simulink model "ROSCO_v1"  (R2023a)
settings: Solver=ode4  StartTime=0.0  StopTime=TMax  FixedStep=simu.dt  RelTol=1e-3  EnableMultiTasking=on
undefined symbols (not defined in the file): Azimuth_list, DiscIntNeverNeededParam, F, n_FixFrameInputs, n_FixFrameOutputs, n_RotTripletInputs, n_RotTripletOutputs, new_seq_inp, new_seq_out, OutList, Parameter, R, rpm2radps, simu, StateSpace, strmatch
libraries: simulink x10
(part 1 of 3)
settings Model: Creator=nabbas  LastModifiedBy=16708
settings SolverCC: AlgebraicLoopSolver=TrustRegion
settings DataIOCC: SaveTime=off  ReturnWorkspaceOutputs=off  SignalLoggingName=sigsOut
settings DebuggingCC: UnconnectedInputMsg=warning  UnconnectedOutputMsg=warning  UnconnectedLineMsg=warning  ArithmeticOperatorsInVariantConditions=warning
settings ModelReferenceCC: EnableRefExpFcnMdlSchedulingChecks=on
settings SFSimCC: SimUseLocalCustomCode=off  CustomCodeUndefinedFunction=UseInterfaceOnly
settings RTWCC: RTWUseLocalCustomCode=off
settings CodeAppCC: StateflowObjectComments=on

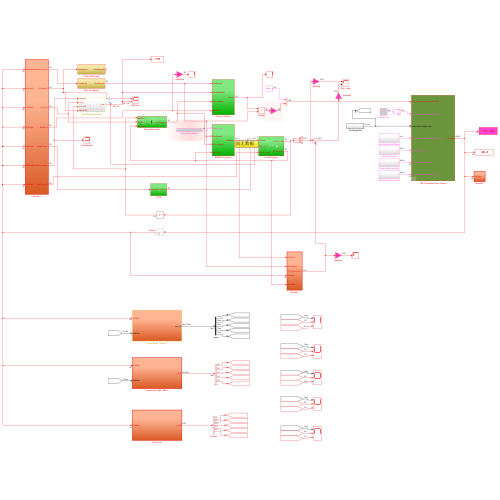
[thumbnail: Simulink's stored preview of the top-level diagram]
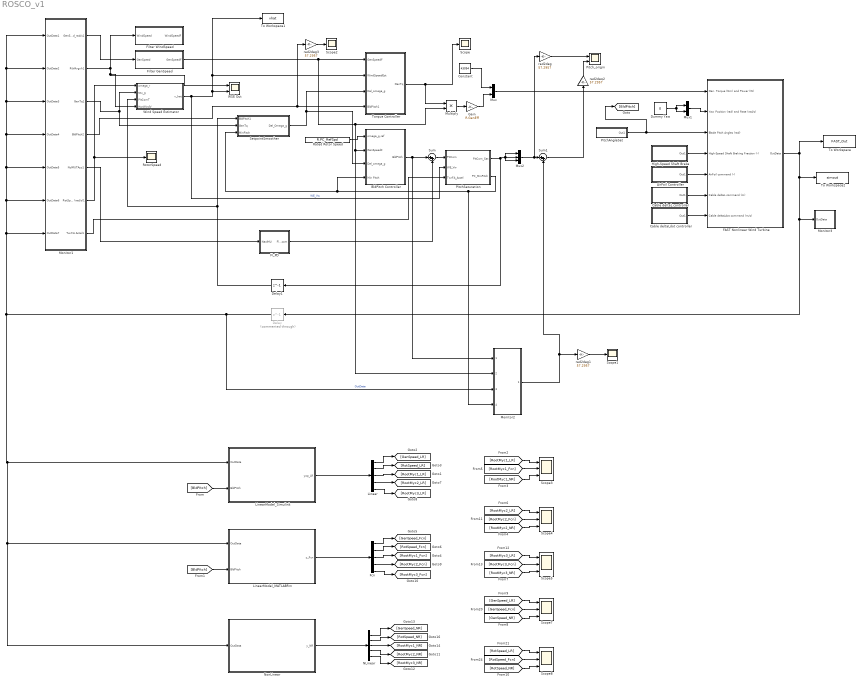
== system ROSCO_v1 ==
  AirFoil Controller : Subsystem
  BldPitch Controller : Subsystem
  Cable deltaL controller : Subsystem
  Cable deltaLdot controller : Subsystem
  Constant : Constant  Value=43094
  Delay : Delay  Commented=through  DelayLength=1
  Delay1 : Delay  DelayLength=1
  Dummy Yaw : Constant  Value=0
  FAST Nonlinear Wind Turbine : Subsystem  mask(FAST Nonlinear Wind Turbine){}
      mask help: This block contains the FAST S-Function.
      mask init:
      | clear FAST_SFunc
  Fcn : Demux  Outputs=5
  Filter GenSpeed : Subsystem
  Filter WindSpeed : Subsystem
  Fl_PD : Subsystem
  Gain : Gain  Gain=R.GenEff
  High-Speed Shaft Brake : Subsystem
  Linear : Demux  Outputs=5
  LinearModel_MATLABFcn : Subsystem  TreatAsAtomicUnit=on
  LinearModel_Simulink : Subsystem  TreatAsAtomicUnit=on
  Monitor1 : Subsystem  TreatAsAtomicUnit=on
  Monitor2 : Subsystem  TreatAsAtomicUnit=on
  Monitor3 : Subsystem  TreatAsAtomicUnit=on
  Multiply : Product
  Mux : Mux  Inputs=2
  Mux1 : Mux  Inputs=2
  Mux2 : Mux  Inputs=3
  NLinear : Demux  Outputs=5
  NonLinear : Subsystem  TreatAsAtomicUnit=on
  PitchAngleSet : Subsystem
  PitchSaturation : Subsystem
  Pitch_origin : Scope  NumInputPorts=2
  Rated Rotor Speed : Constant  Value=R.PC_RefSpd
  RotorSpeed : Scope
  Scope : Scope
  Scope1 : Scope
  Scope2 : Scope
  Scope{3..5,7..8} (5 alike) : Scope  NumInputPorts=3
  SetpointSmoother : Subsystem
  Sum : Sum  Inputs=|++
  Sum1 : Sum  Inputs=|++
  To Workspace : ToWorkspace  VariableName=FAST_Out  SaveFormat=Timeseries  SampleTime=-1
  To Workspace1 : ToWorkspace  VariableName=vhat  SaveFormat=Timeseries  SampleTime=-1
  To Workspace2 : ToWorkspace  VariableName=simout  SaveFormat=Timeseries  SampleTime=-1
  Torque Controller : Subsystem
  WSE Out : Scope  NumInputPorts=2
  Wind Speed Estimator : Subsystem
  rad2deg{,1..3} (4 alike) : Gain  Gain=57.2957
  wires:
  FAST Nonlinear Wind Turbine/1(OutData) -> To Workspace/1, To Workspace2/1, Monitor3/1(OutData), Delay/1
  Dummy Yaw/1 -> Mux1/2, Mux1/1
  Mux1/1 -> FAST Nonlinear Wind Turbine/2(Yaw Position (rad) and Rate (rad/s))
  Multiply/1 -> Gain/1
  Monitor1/1(GenSpeed_rad/s1) -> Filter GenSpeed/1(GenSpeed)
  Torque Controller/1(GenTq) -> Scope/1, Multiply/1
  Monitor1/3(GenTq1) -> Wind Speed Estimator/2(tau_g), SetpointSmoother/2(GenTq)
  SetpointSmoother/1(Del_Omega_g) -> BldPitch Controller/3(Del_omega_g), Torque Controller/3(Del_omega_g)
  Rated Rotor Speed/1 -> BldPitch Controller/1(omega_g,ref)
  Gain/1 -> Mux/2
  Monitor1/2(RtVAvgxh1) -> Filter WindSpeed/1(WindSpeed), Wind Speed Estimator/4(HorWindV), WSE Out/1
  Wind Speed Estimator/1(v_hat) -> PitchSaturation/2(WE_Vw), WSE Out/2, Torque Controller/2(WindSpeedEst), To Workspace1/1  "WE_Vw"
  Delay/1 -> Monitor2/3(OutData), NonLinear/1(OutData), LinearModel_MATLABFcn/1(OutData), LinearModel_Simulink/1(OutData), Monitor1/7(OutData7), Monitor1/6(OutData6), Monitor1/5(OutData5), Monitor1/4(OutData4), Monitor1/3(OutData3), Monitor1/1(OutData1), Monitor1/2(OutData2)  "OutData"
  Monitor1/5(NcIMUTAys1) -> Fl_PD/1(NacIMU)
  Fl_PD/1(Fl_Pitcom) -> Sum/2
  Monitor1/4(BldPitch2) -> rad2deg3/1, Torque Controller/4(BldPitch1)
  Sum/1 -> PitchSaturation/1(PitCom)
  PitchSaturation/1(PitCom_Sat) -> Delay1/1, Mux2/3, Mux2/1, Mux2/2
  PitchSaturation/2(PC_MinPitch) -> Monitor2/4(Min Pitch), BldPitch Controller/4(Min Pitch), SetpointSmoother/3(MinPitch)
  BldPitch Controller/1(BldPitch) -> Monitor2/1(Coll.Pitch), Sum/1
  Monitor1/6(RotSpeed (rad/s)1) -> RotorSpeed/1, Wind Speed Estimator/1(omega_r)
  Delay1/1 -> SetpointSmoother/1(BldPitch1), Wind Speed Estimator/3(PitComT)
  Monitor1/7(TwrFA Accel1) -> PitchSaturation/3(TwrFA_Accel)
  Mux/1 -> FAST Nonlinear Wind Turbine/1(Gen. Torque (Nm) and Power (W))
  Filter GenSpeed/1(GenSpeedF) -> Torque Controller/1(GenSpeedF), Multiply/2, Monitor2/2(Gen Speed), BldPitch Controller/2(GenSpeedF)
  Mux2/1 -> rad2deg/1, Sum1/1
  Sum1/1 -> rad2deg2/1
  High-Speed Shaft Brake/1(Out1) -> FAST Nonlinear Wind Turbine/4(High-Speed Shaft Braking Fraction (-))
  AirFoil Controller/1(Out1) -> FAST Nonlinear Wind Turbine/5(AirFoil command (-))
  Cable deltaL controller/1(Out1) -> FAST Nonlinear Wind Turbine/6(Cable deltaL command (m))
  Cable deltaLdot controller/1(Out1) -> FAST Nonlinear Wind Turbine/7(Cable deltaLdot command (m/s))
  rad2deg/1 -> Pitch_origin/1
  Monitor2/1(IPC Cmd (rad,3)) -> rad2deg1/1, Sum1/2
  rad2deg1/1 -> Scope1/1
  rad2deg2/1 -> Pitch_origin/2
  Constant/1 -> Mux/1
  rad2deg3/1 -> Scope2/1
  [BldPitch] -> LinearModel_Simulink/2(BldPitch)
  [BldPitch] -> LinearModel_MATLABFcn/2(BldPitch)
  LinearModel_Simulink/1(yop_LR) -> Linear/1
  Linear/5 -> [RootMyc3_LR]
  Linear/3 -> [RootMyc1_LR]
  Linear/2 -> [RotSpeed_LR]
  Linear/4 -> [RootMyc2_LR]
  Linear/1 -> [GenSpeed_LR]
  Fcn/4 -> [RootMyc2_Fcn]
  Fcn/1 -> [GenSpeed_Fcn]
  Fcn/3 -> [RootMyc1_Fcn]
  LinearModel_MATLABFcn/1(y_Fcn) -> Fcn/1
  Fcn/5 -> [RootMyc3_Fcn]
  Fcn/2 -> [RotSpeed_Fcn]
  [RootMyc2_LR] -> Scope4/1
  [RootMyc3_Fcn] -> Scope5/2
  [RotSpeed_LR] -> Scope8/1
  [GenSpeed_LR] -> Scope7/1
  [RootMyc2_Fcn] -> Scope4/2
  [GenSpeed_Fcn] -> Scope7/2
  [RootMyc1_Fcn] -> Scope3/2
  [RootMyc3_LR] -> Scope5/1
  [RotSpeed_Fcn] -> Scope8/2
  [RootMyc1_LR] -> Scope3/1
  NLinear/3 -> [RootMyc1_NR]
  NonLinear/1(y_NR) -> NLinear/1
  NLinear/5 -> [RootMyc3_NR]
  NLinear/2 -> [RotSpeed_NR]
  NLinear/4 -> [RootMyc2_NR]
  NLinear/1 -> [GenSpeed_NR]
  [RootMyc1_NR] -> Scope3/3
  [RootMyc2_NR] -> Scope4/3
  [RootMyc3_NR] -> Scope5/3
  [GenSpeed_NR] -> Scope7/3
  [RotSpeed_NR] -> Scope8/3
  PitchAngleSet/1(Out1) -> [BldPitch], FAST Nonlinear Wind Turbine/3(Blade Pitch Angles (rad))

== system ROSCO_v1/AirFoil Controller ==
  Airfoil command : Constant  Value=zeros(1,3)'
  Out1 : Outport
  wires:
  Airfoil command/1 -> Out1/1

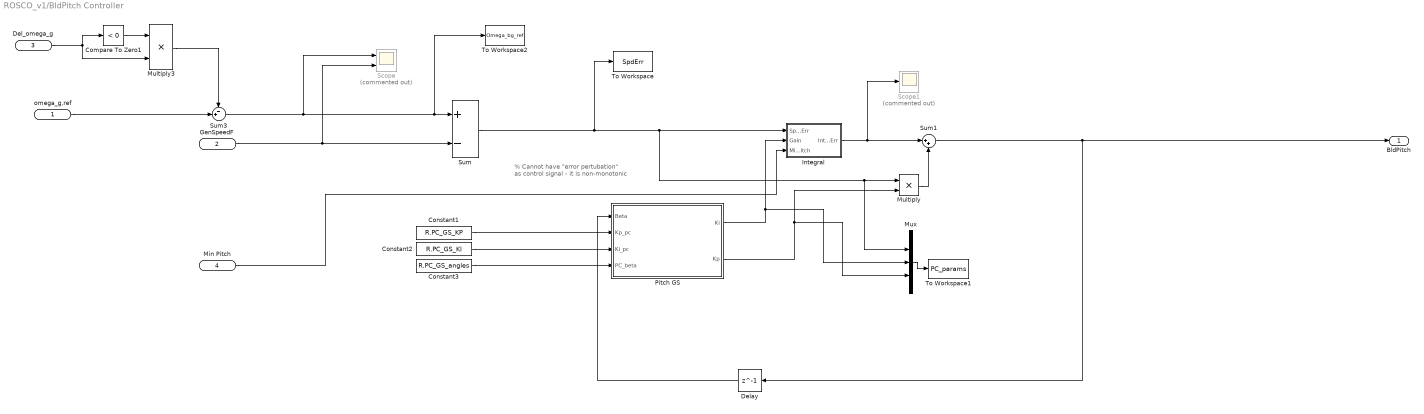
== system ROSCO_v1/BldPitch Controller ==
  note: % Cannot have "error pertubation" as control signal
      | - it is non-monotonic
  omega_g,ref : Inport
  GenSpeedF : Inport  Port=2
  Del_omega_g : Inport  Port=3
  Min Pitch : Inport  Port=4
  Compare To Zero1 : simulink/Logic and Bit Operations/Compare To Zero  relop=<  OutDataTypeStr=boolean
  Constant1 : Constant  Value=R.PC_GS_KP
  Constant2 : Constant  Value=R.PC_GS_KI
  Constant3 : Constant  Value=R.PC_GS_angles
  Delay : Delay  DelayLength=1
  Integral : Subsystem
  Multiply : Product
  Multiply3 : Product
  Mux : Mux  Inputs=5
  Pitch GS : MATLAB Function  TreatAsAtomicUnit=on
  Scope : Scope  Commented=on  NumInputPorts=2
  Scope1 : Scope  Commented=on
  Sum : Sum  Inputs=+-
  Sum1 : Sum  Inputs=|++
  Sum3 : Sum  Inputs=-+|
  To Workspace : ToWorkspace  VariableName=SpdErr  SaveFormat=Timeseries  SampleTime=-1
  To Workspace1 : ToWorkspace  VariableName=PC_params  SaveFormat=Structure  SampleTime=-1
  To Workspace2 : ToWorkspace  VariableName=Omega_bg_ref  SaveFormat=Timeseries  SampleTime=-1
  BldPitch : Outport  VectorParamsAs1DForOutWhenUnconnected=off
  wires:
  Multiply/1 -> Sum1/2
  Integral/1(IntSpdErr) -> Scope1/1, Sum1/1
  Pitch GS/1(Ki) -> Mux/3, Integral/2(Gain)
  Pitch GS/2(Kp) -> Mux/4, Multiply/2
  Mux/1 -> To Workspace1/1
  Sum1/1 -> Delay/1, BldPitch/1
  Sum3/1 -> Scope/1, To Workspace2/1, Sum/1
  GenSpeedF/1 -> Scope/2, Sum/2
  Compare To Zero1/1 -> Multiply3/1
  Del_omega_g/1 -> Compare To Zero1/1, Multiply3/2
  Multiply3/1 -> Sum3/1
  omega_g,ref/1 -> Sum3/2
  Constant1/1 -> Pitch GS/2(Kp_pc)
  Constant2/1 -> Pitch GS/3(Ki_pc)
  Constant3/1 -> Pitch GS/4(PC_beta)
  Delay/1 -> Pitch GS/1(Beta)
  Min Pitch/1 -> Integral/3(Min Pitch)
  Sum/1 -> To Workspace/1, Mux/2, Multiply/1, Integral/1(SpeedErr)

== system ROSCO_v1/Cable deltaL controller ==
  Cable deltaL command : Constant  Value=zeros(1,20)'
  Out1 : Outport
  wires:
  Cable deltaL command/1 -> Out1/1

== system ROSCO_v1/Cable deltaLdot controller ==
  Cable deltaLdot command : Constant  Value=zeros(1,20)'
  Out1 : Outport
  wires:
  Cable deltaLdot command/1 -> Out1/1

== system ROSCO_v1/FAST Nonlinear Wind Turbine ==
  Gen. Torque (Nm) and Power (W) : Inport
  Yaw Position (rad) and Rate (rad/s) : Inport  Port=2
  Blade Pitch Angles (rad) : Inport  Port=3
  High-Speed Shaft Braking Fraction (-) : Inport  Port=4
  AirFoil command (-) : Inport  Port=5
  Cable deltaL command (m) : Inport  Port=6
  Cable deltaLdot command (m/s) : Inport  Port=7
  Mux1 : Mux  Inputs=7
  S-Function : S-Function  FunctionName=FAST_SFunc  Parameters=FAST_InputFileName, TMax, 0  SFunctionDeploymentMode=off  EnableBusSupport=off
  Signal Specification1 : SignalSpecification  OutDataTypeStr=double  Dimensions=2
  Signal Specification2 : SignalSpecification  OutDataTypeStr=double  Dimensions=2
  OutData : Outport
  wires:
  Gen. Torque (Nm) and Power (W)/1 -> Signal Specification1/1
  S-Function/1 -> OutData/1
  Mux1/1 -> S-Function/1
  Blade Pitch Angles (rad)/1 -> Mux1/3
  Yaw Position (rad) and Rate (rad/s)/1 -> Signal Specification2/1
  Signal Specification1/1 -> Mux1/1
  Signal Specification2/1 -> Mux1/2
  High-Speed Shaft Braking Fraction (-)/1 -> Mux1/4
  AirFoil command (-)/1 -> Mux1/5
  Cable deltaL command (m)/1 -> Mux1/6
  Cable deltaLdot command (m/s)/1 -> Mux1/7

== system ROSCO_v1/Filter GenSpeed ==
  GenSpeed : Inport
  Discrete Filter : DiscreteFilter  Numerator=F.HSS.b  Denominator=F.HSS.a  InitialStates=R.VS_RefSpd/(sum(F.HSS.a(2:end))+1)
  Scope : Scope  NumInputPorts=2
  To Workspace2 : ToWorkspace  VariableName=Om_f  SaveFormat=Timeseries  SampleTime=-1
  GenSpeedF : Outport  VectorParamsAs1DForOutWhenUnconnected=off
  wires:
  Discrete Filter/1 -> Scope/2, To Workspace2/1, GenSpeedF/1
  GenSpeed/1 -> Scope/1, Discrete Filter/1

== system ROSCO_v1/Filter WindSpeed ==
  WindSpeed : Inport
  Discrete Filter : DiscreteFilter  Numerator=F.Wind.b  Denominator=F.Wind.a  InitialStates=10
  To Workspace2 : ToWorkspace  VariableName=WindSpeedF  SaveFormat=Timeseries  SampleTime=-1
  WindSpeedF : Outport  VectorParamsAs1DForOutWhenUnconnected=off
  wires:
  Discrete Filter/1 -> WindSpeedF/1, To Workspace2/1
  WindSpeed/1 -> Discrete Filter/1

== system ROSCO_v1/Fl_PD ==
  NacIMU : Inport
  Constant : Constant
  Enable : Gain  Gain=R.Fl_Mode
  Fl_HPF : DiscreteFilter  Numerator=F.F_Fl_HPF.b  Denominator=F.F_Fl_HPF.b
  Fl_LPF : DiscreteFilter  Numerator=F.F_Fl.b  Denominator=F.F_Fl.a
  Gain1 : Gain  Gain=-R.Fl_Kp
  Integral : Subsystem
  Scope : Scope
  Fl_Pitcom : Outport
  wires:
  Constant/1 -> Integral/2(Gain)
  NacIMU/1 -> Fl_LPF/1  "FA_AccR"
  Integral/1(Int x) -> Gain1/1
  Fl_HPF/1 -> Integral/1(x)  "FA_AccF"
  Gain1/1 -> Enable/1  "Fl_Pitcom"
  Enable/1 -> Scope/1, Fl_Pitcom/1  "Fl_Pitcom"
  Fl_LPF/1 -> Fl_HPF/1  "FA_AccF"

== system ROSCO_v1/High-Speed Shaft Brake ==
  High-Speed Shaft Braking Fraction : Constant  Value=0
  Out1 : Outport
  wires:
  High-Speed Shaft Braking Fraction/1 -> Out1/1

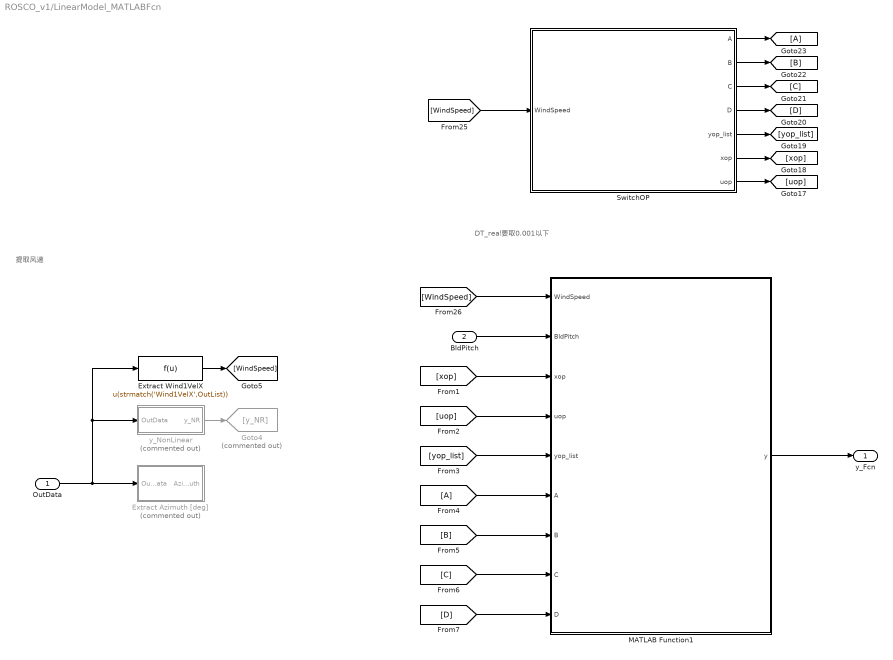
== system ROSCO_v1/LinearModel_MATLABFcn ==
  note: DT_real要取0.001以下
  note: 提取风速
  OutData : Inport
  BldPitch : Inport  Port=2
  Extract Azimuth [deg] : Subsystem  Commented=on
  Extract Wind1VelX : Fcn  Expr=u(strmatch('Wind1VelX',OutList))
  From4 : From
  Goto23 : Goto
  Goto4 : Goto  Commented=on  GotoTag=y_NR
  MATLAB Function1 : MATLAB Function  TreatAsAtomicUnit=on
  SwitchOP : Subsystem
  y_NonLinear : Subsystem  Commented=on
  y_Fcn : Outport
  wires:
  Extract Wind1VelX/1 -> [WindSpeed]
  y_NonLinear/1(y_NR) -> Goto4/1
  OutData/1 -> Extract Azimuth [deg]/1(OutData), y_NonLinear/1(OutData), Extract Wind1VelX/1
  BldPitch/1 -> MATLAB Function1/2(BldPitch)
  [WindSpeed] -> MATLAB Function1/1(WindSpeed)
  [xop] -> MATLAB Function1/3(xop)
  [uop] -> MATLAB Function1/4(uop)
  [yop_list] -> MATLAB Function1/5(yop_list)
  From4/1 -> MATLAB Function1/6(A)
  [B] -> MATLAB Function1/7(B)
  [C] -> MATLAB Function1/8(C)
  [D] -> MATLAB Function1/9(D)
  MATLAB Function1/1(y) -> y_Fcn/1
  SwitchOP/2(B) -> [B]
  SwitchOP/3(C) -> [C]
  SwitchOP/5(yop_list) -> [yop_list]
  SwitchOP/4(D) -> [D]
  SwitchOP/7(uop) -> [uop]
  SwitchOP/1(A) -> Goto23/1
  SwitchOP/6(xop) -> [xop]
  [WindSpeed] -> SwitchOP/1(WindSpeed)

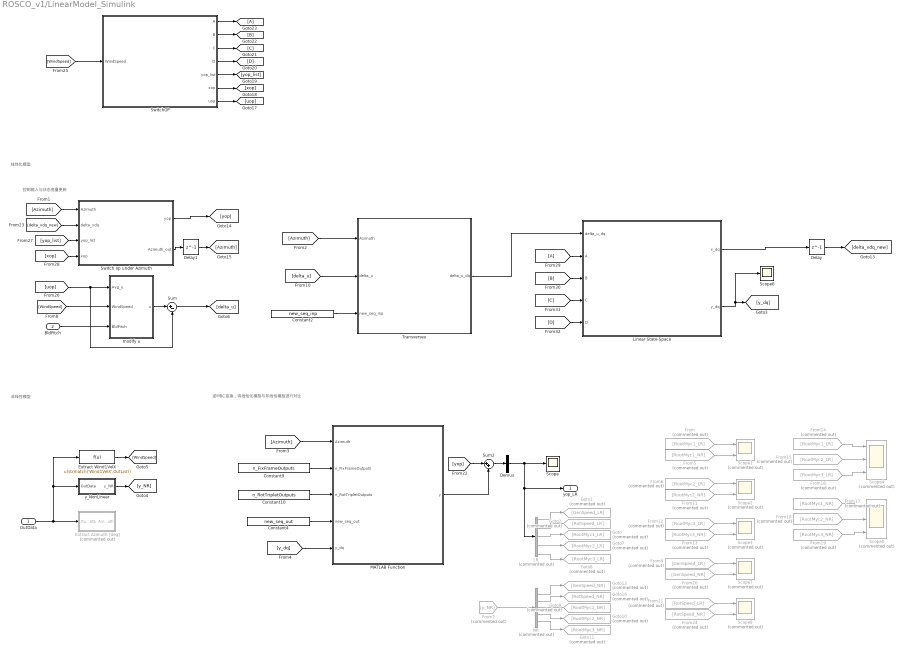
== system ROSCO_v1/LinearModel_Simulink ==
  note: 逆MBC变换，将线性化模型与非线性模型进行对比
  note: 控制输入与状态变量更新
  note: 线性化模型
  note: 非线性模型
  OutData : Inport
  BldPitch : Inport  Port=2
  Constant10 : Constant  Value=n_RotTripletOutputs
  Constant2 : Constant  Value=new_seq_inp
  Constant4 : Constant  Value=new_seq_out
  Constant9 : Constant  Value=n_FixFrameOutputs
  Delay : Delay  DelayLength=1  InitialCondition=0
  Delay1 : Delay  DelayLength=1  InitialCondition=0
  Demux : Demux  Outputs=1
  Extract Azimuth [deg] : Subsystem  Commented=on
  Extract Wind1VelX : Fcn  Expr=u(strmatch('Wind1VelX',OutList))
  From : From  Commented=on  GotoTag=RootMyc1_LR
  From11 : From  Commented=on  GotoTag=RootMyc2_NR
  From12 : From  Commented=on  GotoTag=RootMyc3_LR
  From13 : From  Commented=on  GotoTag=RootMyc3_NR
  From14 : From  Commented=on  GotoTag=RootMyc1_LR
  From15 : From  Commented=on  GotoTag=RootMyc2_LR
  From16 : From  Commented=on  GotoTag=RootMyc3_LR
  From17 : From  Commented=on  GotoTag=RootMyc1_NR
  From18 : From  Commented=on  GotoTag=RootMyc2_NR
  From19 : From  Commented=on  GotoTag=RootMyc3_NR
  From20 : From  Commented=on  GotoTag=GenSpeed_NR
  From21 : From  Commented=on  GotoTag=RotSpeed_LR
  From24 : From  Commented=on  GotoTag=RotSpeed_NR
  From29 : From
  From5 : From  Commented=on  GotoTag=RootMyc1_NR
  From6 : From  Commented=on  GotoTag=RootMyc2_LR
  From7 : From  Commented=on  GotoTag=y_NR
  From9 : From  Commented=on  GotoTag=GenSpeed_LR
  Goto : Goto  Commented=on  GotoTag=RootMyc1_LR
  Goto1 : Goto  Commented=on  GotoTag=GenSpeed_LR
  Goto10 : Goto  Commented=on  GotoTag=RootMyc2_NR
  Goto11 : Goto  Commented=on  GotoTag=RootMyc3_NR
  Goto12 : Goto  Commented=on  GotoTag=GenSpeed_NR
  Goto16 : Goto  Commented=on  GotoTag=RotSpeed_NR
  Goto2 : Goto  Commented=on  GotoTag=RotSpeed_LR
  Goto23 : Goto
  Goto7 : Goto  Commented=on  GotoTag=RootMyc2_LR
  Goto8 : Goto  Commented=on  GotoTag=RootMyc3_LR
  Goto9 : Goto  Commented=on  GotoTag=RootMyc1_NR
  LR : Demux  Commented=on  Outputs=5
  Linear State-Space : Subsystem
  MATLAB Function : MATLAB Function  TreatAsAtomicUnit=on
  NR : Demux  Commented=on  Outputs=5
  Scope : Scope
  Scope{1..3,7..8} (5 alike) : Scope  Commented=on  NumInputPorts=2
  Scope4 : Scope  Commented=on  NumInputPorts=3
  Scope5 : Scope  Commented=on  NumInputPorts=3
  Scope6 : Scope
  Sum : Sum  Inputs=|+-
  Sum2 : Sum  Inputs=|++
  Switch op under Azimuth : Subsystem
  SwitchOP : Subsystem
  Transverseu : Subsystem
  modify u : MATLAB Function  TreatAsAtomicUnit=on
  y_NonLinear : Subsystem
  yop_LR : Outport
  wires:
  OutData/1 -> Extract Wind1VelX/1, y_NonLinear/1(OutData), Extract Azimuth [deg]/1(OutData)
  Transverseu/1(delta_u_dq) -> Linear State-Space/1(delta_u_dq)
  Demux/1 -> Scope/1, yop_LR/1, LR/1
  y_NonLinear/1(y_NR) -> [y_NR]
  From7/1 -> NR/1
  Extract Wind1VelX/1 -> [WindSpeed]
  [Azimuth] -> Transverseu/1(Azimuth)
  Sum/1 -> [delta_u]
  [WindSpeed] -> modify u/2(WindSpeed)
  [uop] -> Sum/2, modify u/1(Avg_u)
  modify u/1(u) -> Sum/1
  [delta_u] -> Transverseu/2(delta_u)
  Constant2/1 -> Transverseu/3(new_seq_inp)
  Constant9/1 -> MATLAB Function/2(n_FixFrameOutputs)
  Constant10/1 -> MATLAB Function/3(n_RotTripletOutputs)
  [Azimuth] -> MATLAB Function/1(Azimuth)
  Constant4/1 -> MATLAB Function/4(new_seq_out)
  [y_dq] -> MATLAB Function/5(y_dq)
  LR/3 -> Goto/1
  LR/4 -> Goto7/1
  LR/5 -> Goto8/1
  NR/3 -> Goto9/1
  NR/4 -> Goto10/1
  NR/5 -> Goto11/1
  From/1 -> Scope1/1
  From5/1 -> Scope1/2
  From6/1 -> Scope2/1
  From11/1 -> Scope2/2
  From12/1 -> Scope3/1
  From13/1 -> Scope3/2
  From14/1 -> Scope4/1
  From15/1 -> Scope4/2
  From16/1 -> Scope4/3
  From17/1 -> Scope5/1
  From18/1 -> Scope5/2
  From19/1 -> Scope5/3
  Linear State-Space/1(x_dq) -> Delay/1
  Switch op under Azimuth/1(yop) -> [yop]
  [Azimuth] -> Switch op under Azimuth/1(Azimuth)
  [yop] -> Sum2/1
  Sum2/1 -> Demux/1
  Linear State-Space/2(y_dq) -> Scope6/1, [y_dq]
  MATLAB Function/1(y) -> Sum2/2
  Delay/1 -> [delta_xdq_new]
  Switch op under Azimuth/2(Azimuth_out) -> Delay1/1
  Delay1/1 -> [Azimuth]
  [delta_xdq_new] -> Switch op under Azimuth/2(delta_xdq)
  LR/1 -> Goto1/1
  LR/2 -> Goto2/1
  NR/1 -> Goto12/1
  NR/2 -> Goto16/1
  From9/1 -> Scope7/1
  From20/1 -> Scope7/2
  From21/1 -> Scope8/1
  From24/1 -> Scope8/2
  BldPitch/1 -> modify u/3(BldPitch)
  [WindSpeed] -> SwitchOP/1(WindSpeed)
  SwitchOP/7(uop) -> [uop]
  SwitchOP/6(xop) -> [xop]
  SwitchOP/5(yop_list) -> [yop_list]
  SwitchOP/4(D) -> [D]
  SwitchOP/3(C) -> [C]
  SwitchOP/2(B) -> [B]
  SwitchOP/1(A) -> Goto23/1
  [yop_list] -> Switch op under Azimuth/3(yop_list)
  [xop] -> Switch op under Azimuth/4(xop)
  From29/1 -> Linear State-Space/2(A)
  [B] -> Linear State-Space/3(B)
  [C] -> Linear State-Space/4(C)
  [D] -> Linear State-Space/5(D)

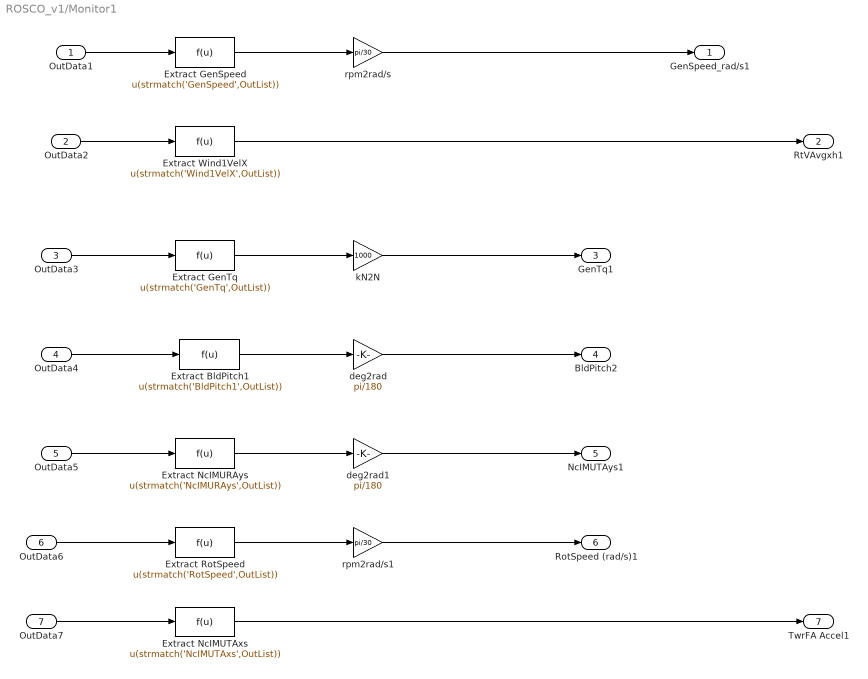
== system ROSCO_v1/Monitor1 ==
  OutData1 : Inport
  OutData2 : Inport  Port=2
  OutData3 : Inport  Port=3
  OutData4 : Inport  Port=4
  OutData5 : Inport  Port=5
  OutData6 : Inport  Port=6
  OutData7 : Inport  Port=7
  Extract BldPitch1 : Fcn  Expr=u(strmatch('BldPitch1',OutList))
  Extract GenSpeed : Fcn  Expr=u(strmatch('GenSpeed',OutList))
  Extract GenTq : Fcn  Expr=u(strmatch('GenTq',OutList))
  Extract NcIMURAys : Fcn  Expr=u(strmatch('NcIMURAys',OutList))
  Extract NcIMUTAxs : Fcn  Expr=u(strmatch('NcIMUTAxs',OutList))
  Extract RotSpeed : Fcn  Expr=u(strmatch('RotSpeed',OutList))
  Extract Wind1VelX : Fcn  Expr=u(strmatch('Wind1VelX',OutList))
  deg2rad : Gain  Gain=pi/180
  deg2rad1 : Gain  Gain=pi/180
  kN2N : Gain  Gain=1000
  rpm2rad/s : Gain  Gain=pi/30
  rpm2rad/s1 : Gain  Gain=pi/30
  GenSpeed_rad/s1 : Outport  VectorParamsAs1DForOutWhenUnconnected=off
  RtVAvgxh1 : Outport  Port=2  VectorParamsAs1DForOutWhenUnconnected=off
  GenTq1 : Outport  Port=3  VectorParamsAs1DForOutWhenUnconnected=off
  BldPitch2 : Outport  Port=4  VectorParamsAs1DForOutWhenUnconnected=off
  NcIMUTAys1 : Outport  Port=5  VectorParamsAs1DForOutWhenUnconnected=off
  RotSpeed (rad/s)1 : Outport  Port=6  VectorParamsAs1DForOutWhenUnconnected=off
  TwrFA Accel1 : Outport  Port=7  VectorParamsAs1DForOutWhenUnconnected=off
  wires:
  Extract NcIMURAys/1 -> deg2rad1/1
  Extract GenSpeed/1 -> rpm2rad/s/1
  OutData5/1 -> Extract NcIMURAys/1
  Extract NcIMUTAxs/1 -> TwrFA Accel1/1
  rpm2rad/s1/1 -> RotSpeed (rad/s)1/1
  Extract RotSpeed/1 -> rpm2rad/s1/1
  Extract BldPitch1/1 -> deg2rad/1
  OutData4/1 -> Extract BldPitch1/1
  rpm2rad/s/1 -> GenSpeed_rad/s1/1
  OutData3/1 -> Extract GenTq/1
  deg2rad1/1 -> NcIMUTAys1/1
  kN2N/1 -> GenTq1/1
  OutData7/1 -> Extract NcIMUTAxs/1
  deg2rad/1 -> BldPitch2/1
  OutData2/1 -> Extract Wind1VelX/1
  Extract GenTq/1 -> kN2N/1
  Extract Wind1VelX/1 -> RtVAvgxh1/1
  OutData1/1 -> Extract GenSpeed/1
  OutData6/1 -> Extract RotSpeed/1

== system ROSCO_v1/Monitor2 ==
  Coll.Pitch : Inport
  Gen Speed : Inport  Port=2
  OutData : Inport  Port=3
  Min Pitch : Inport  Port=4
  Cyclic Pitch controller : Subsystem  TreatAsAtomicUnit=on
      settings: MinAlgLoopOccurrences=on
  IPC Cmd (rad,3) : Outport
  wires:
  Min Pitch/1 -> Cyclic Pitch controller/4(Min PItch (rad))
  Coll.Pitch/1 -> Cyclic Pitch controller/1(Coll. Pitch)
  Cyclic Pitch controller/1(IPC Cmd (rad,3)) -> IPC Cmd (rad,3)/1
  Gen Speed/1 -> Cyclic Pitch controller/2(Gen Speed)
  OutData/1 -> Cyclic Pitch controller/3(OutData)

== system ROSCO_v1/Monitor3 ==
  OutData : Inport
  Extract BldPitch1 : Fcn  Expr=u(strmatch('BldPitch1',OutList))
  Extract GenPwr : Fcn  Expr=u(strmatch('GenPwr',OutList))
  Extract GenTq : Fcn  Expr=u(strmatch('GenTq',OutList))
  Extract RotSpeed : Fcn  Expr=u(strmatch('RotSpeed',OutList))
  Scope : Scope  NumInputPorts=4
  wires:
  OutData/1 -> Extract RotSpeed/1, Extract GenPwr/1, Extract BldPitch1/1, Extract GenTq/1
  Extract GenPwr/1 -> Scope/4
  Extract GenTq/1 -> Scope/2
  Extract BldPitch1/1 -> Scope/3
  Extract RotSpeed/1 -> Scope/1

== system ROSCO_v1/NonLinear ==
  OutData : Inport
  Extract GenSpeed : Fcn  Expr=u(strmatch('GenSpeed',OutList))
  Extract RootMyc1 : Fcn  Expr=u(strmatch('RootMyc1',OutList))
  Extract RootMyc2 : Fcn  Expr=u(strmatch('RootMyc2',OutList))
  Extract RootMyc3 : Fcn  Expr=u(strmatch('RootMyc3',OutList))
  Extract RotSpeed : Fcn  Expr=u(strmatch('RotSpeed',OutList))
  Mux : Mux  Inputs=5
  y_NR : Outport
  wires:
  Extract RotSpeed/1 -> Mux/2
  Extract GenSpeed/1 -> Mux/1
  Mux/1 -> y_NR/1
  OutData/1 -> Extract GenSpeed/1, Extract RotSpeed/1, Extract RootMyc2/1, Extract RootMyc3/1, Extract RootMyc1/1
  Extract RootMyc1/1 -> Mux/3
  Extract RootMyc2/1 -> Mux/4
  Extract RootMyc3/1 -> Mux/5

== system ROSCO_v1/PitchAngleSet ==
  Blade Pitch Angles [deg] : Constant  Value=8.42
  Blade Pitch Angles [deg]1 : Constant  Value=8.42
  Blade Pitch Angles [deg]2 : Constant  Value=8.42
  Mux3 : Mux  Inputs=3
  Step : Step  Time=100  After=0  SampleTime=0
  Step1 : Step  Time=100  After=0  SampleTime=0
  Step2 : Step  Time=100  After=0  SampleTime=0
  Sum1 : Sum  Inputs=|++
  Sum2 : Sum  Inputs=|++
  Sum3 : Sum  Inputs=|++
  deg2rad : Gain  Gain=1/(57.2957)
  deg2rad1 : Gain  Gain=1/(57.2957)
  deg2rad2 : Gain  Gain=1/(57.2957)
  Out1 : Outport
  wires:
  Blade Pitch Angles [deg]/1 -> Sum2/1
  Sum2/1 -> deg2rad/1
  Mux3/1 -> Out1/1
  Step/1 -> Sum2/2
  deg2rad/1 -> Mux3/1
  Sum1/1 -> deg2rad1/1
  deg2rad1/1 -> Mux3/2
  Blade Pitch Angles [deg]1/1 -> Sum1/1
  Step1/1 -> Sum1/2
  Sum3/1 -> deg2rad2/1
  deg2rad2/1 -> Mux3/3
  Blade Pitch Angles [deg]2/1 -> Sum3/1
  Step2/1 -> Sum3/2

== system ROSCO_v1/PitchSaturation ==
  note: 输出桨距角下限
  note: 根据等效风速确定桨距角下限
  PitCom : Inport
  WE_Vw : Inport  Port=2
  TwrFA_Accel : Inport  Port=3
  1-D Lookup Table : Lookup_n-D  NumberOfTableDimensions=1  BreakpointsForDimension1=R.PS_WindSpeeds  Table=R.PS_BldPitchMin  InternalRulePriority=Speed  RndMeth=Simplest
  Constant : Constant  Value=R.PS_Mode
  Constant1 : Constant  Value=R.PC_MinPit
  Constant2 : Constant
  Constant4 : Constant  Value=R.PC_MaxPit
  Discrete Filter : DiscreteFilter  Numerator=F.F_PS.b  Denominator=F.F_PS.a  InitialStates=R.WE_v0/(sum(F.F_PS.a(2:end))+1)
  Integral : Subsystem
  Mux : Mux  Inputs=2
  Rate Limiter1 : RateLimiter  RisingSlewLimit=R.PC_MaxRat  FallingSlewLimit=-R.PC_MaxRat  SampleTimeMode=inherited
  Scope : Scope  Commented=on  NumInputPorts=3
  Scope1 : Scope  Commented=on  NumInputPorts=3
  Sum : Sum  Inputs=|++
  Switch : Switch  Criteria=u2 > Threshold  Threshold=0.5  SaturateOnIntegerOverflow=off  InputSameDT=off
  Variable Saturator1 : MATLAB Function  TreatAsAtomicUnit=on
  PitCom_Sat : Outport
  PC_MinPitch : Outport  Port=2
  wires:
  1-D Lookup Table/1 -> Scope/3, Switch/1
  Constant/1 -> Switch/2
  Discrete Filter/1 -> Scope/2, 1-D Lookup Table/1  "Vhatf"
  Constant1/1 -> Switch/3
  Switch/1 -> PC_MinPitch/1, Variable Saturator1/2(lowerLimit)  "PC_MinPit"
  Constant4/1 -> Variable Saturator1/3(upperLimit)
  Variable Saturator1/1(pitchCommandOut) -> Scope1/1, Rate Limiter1/1
  Rate Limiter1/1 -> Scope1/2, PitCom_Sat/1
  PitCom/1 -> Variable Saturator1/1(pitchCommand)
  TwrFA_Accel/1 -> Integral/1(x)
  Constant2/1 -> Integral/2(Gain)
  WE_Vw/1 -> Mux/1, Sum/1
  Sum/1 -> Mux/2, Discrete Filter/1
  Mux/1 -> Scope/1

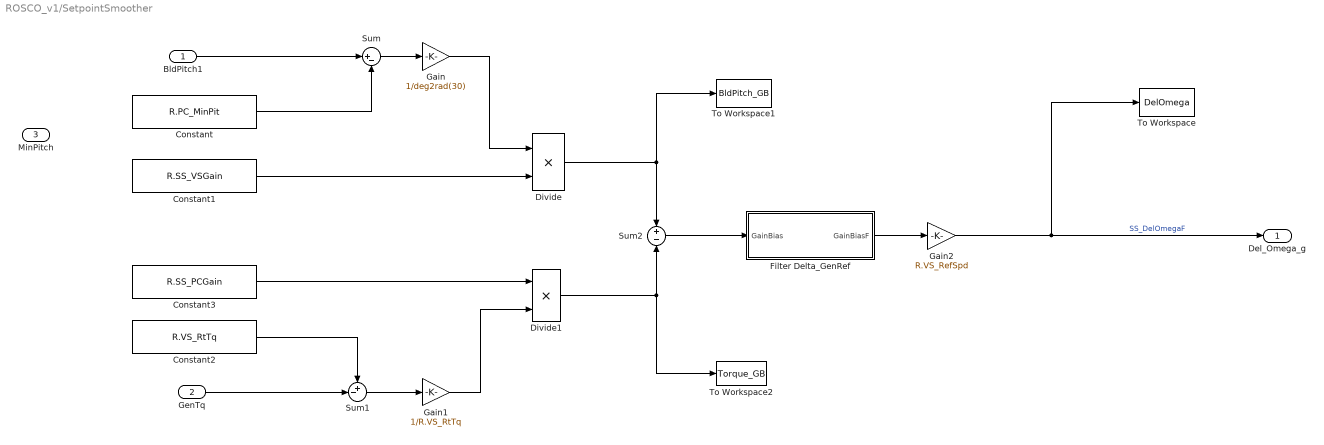
== system ROSCO_v1/SetpointSmoother ==
  BldPitch1 : Inport
  GenTq : Inport  Port=2
  MinPitch : Inport  Port=3
  Constant : Constant  Value=R.PC_MinPit
  Constant1 : Constant  Value=R.SS_VSGain
  Constant2 : Constant  Value=R.VS_RtTq
  Constant3 : Constant  Value=R.SS_PCGain
  Divide : Product  Inputs=**
  Divide1 : Product  Inputs=**
  Filter Delta_GenRef : Subsystem
  Gain : Gain  Gain=1/deg2rad(30)
  Gain1 : Gain  Gain=1/R.VS_RtTq
  Gain2 : Gain  Gain=R.VS_RefSpd
  Sum : Sum  Inputs=|+-
  Sum1 : Sum  Inputs=+-|
  Sum2 : Sum  Inputs=+|-
  To Workspace : ToWorkspace  VariableName=DelOmega  SaveFormat=Timeseries  SampleTime=-1
  To Workspace1 : ToWorkspace  VariableName=BldPitch_GB  SaveFormat=Timeseries  SampleTime=-1
  To Workspace2 : ToWorkspace  VariableName=Torque_GB  SaveFormat=Timeseries  SampleTime=-1
  Del_Omega_g : Outport  VectorParamsAs1DForOutWhenUnconnected=off
  wires:
  Divide1/1 -> Sum2/2, To Workspace2/1
  Divide/1 -> Sum2/1, To Workspace1/1
  Filter Delta_GenRef/1(GainBiasF) -> Gain2/1
  Constant3/1 -> Divide1/1
  Constant1/1 -> Divide/2
  Sum/1 -> Gain/1
  BldPitch1/1 -> Sum/1
  Sum2/1 -> Filter Delta_GenRef/1(GainBias)
  Constant2/1 -> Sum1/1
  Sum1/1 -> Gain1/1
  GenTq/1 -> Sum1/2
  Gain/1 -> Divide/1
  Gain1/1 -> Divide1/2
  Gain2/1 -> To Workspace/1, Del_Omega_g/1  "SS_DelOmegaF"
  Constant/1 -> Sum/2

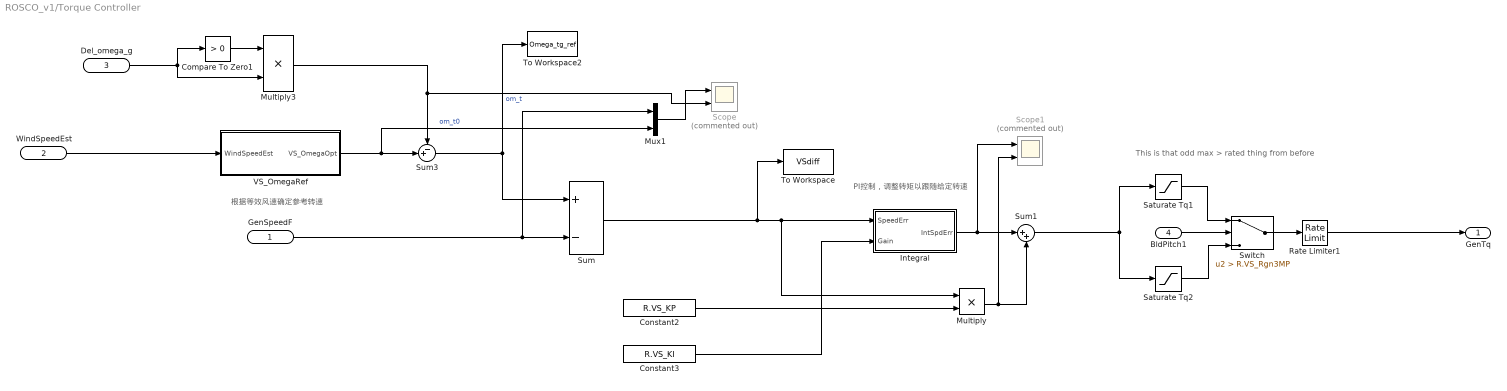
== system ROSCO_v1/Torque Controller ==
  note: PI控制，调整转矩以跟随给定转速
  note: 根据等效风速确定参考转速
  note: This is that odd max > rated thing from before
  GenSpeedF : Inport
  WindSpeedEst : Inport  Port=2
  Del_omega_g : Inport  Port=3
  BldPitch1 : Inport  Port=4
  Compare To Zero1 : simulink/Logic and Bit Operations/Compare To Zero  relop=>  OutDataTypeStr=boolean
  Constant2 : Constant  Value=R.VS_KP
  Constant3 : Constant  Value=R.VS_KI
  Integral : Subsystem
  Multiply : Product
  Multiply3 : Product
  Mux1 : Mux  Inputs=2
  Rate Limiter1 : RateLimiter  RisingSlewLimit=R.VS_MaxRat  FallingSlewLimit=-R.VS_MaxRat  SampleTimeMode=inherited  InitialCondition=R.VS_RtTq
  Saturate Tq1 : Saturate  UpperLimit=R.VS_RtTq  LowerLimit=0
  Saturate Tq2 : Saturate  UpperLimit=R.VS_RtTq  LowerLimit=0
  Scope : Scope  Commented=on  NumInputPorts=2
  Scope1 : Scope  Commented=on  NumInputPorts=2
  Sum : Sum  Inputs=+-
  Sum1 : Sum  Inputs=|++
  Sum3 : Sum  Inputs=-+|
  Switch : Switch  Criteria=u2 > Threshold  Threshold=R.VS_Rgn3MP  SaturateOnIntegerOverflow=off  InputSameDT=off
  To Workspace : ToWorkspace  VariableName=VSdiff  SaveFormat=Timeseries  SampleTime=-1
  To Workspace2 : ToWorkspace  VariableName=Omega_tg_ref  SaveFormat=Timeseries  SampleTime=-1
  VS_OmegaRef : Subsystem
  GenTq : Outport  VectorParamsAs1DForOutWhenUnconnected=off
  wires:
  Multiply/1 -> Scope1/2, Sum1/2
  Integral/1(IntSpdErr) -> Scope1/1, Sum1/1
  Constant2/1 -> Multiply/2
  Constant3/1 -> Integral/2(Gain)
  VS_OmegaRef/1(VS_OmegaOpt) -> Mux1/2, Sum3/2  "om_t0"
  GenSpeedF/1 -> Mux1/1, Sum/2
  Sum3/1 -> To Workspace2/1, Sum/1  "om_t"
  Saturate Tq2/1 -> Switch/3
  Switch/1 -> Rate Limiter1/1
  Saturate Tq1/1 -> Switch/1
  BldPitch1/1 -> Switch/2
  Compare To Zero1/1 -> Multiply3/1
  Del_omega_g/1 -> Compare To Zero1/1, Multiply3/2
  Multiply3/1 -> Scope/2, Sum3/1
  Mux1/1 -> Scope/1
  Sum1/1 -> Saturate Tq2/1, Saturate Tq1/1
  Rate Limiter1/1 -> GenTq/1
  Sum/1 -> To Workspace/1, Integral/1(SpeedErr), Multiply/1
  WindSpeedEst/1 -> VS_OmegaRef/1(WindSpeedEst)

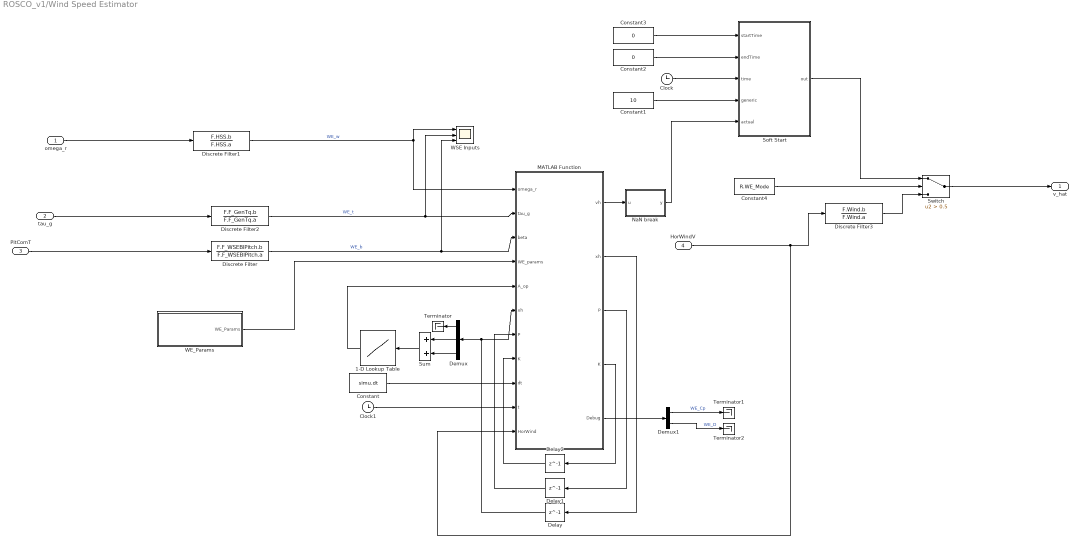
== system ROSCO_v1/Wind Speed Estimator ==
  omega_r : Inport
  tau_g : Inport  Port=2
  PitComT : Inport  Port=3
  HorWindV : Inport  Port=4
  1-D Lookup Table : Lookup_n-D  NumberOfTableDimensions=1  BreakpointsForDimension1=[-5:5]  Table=tanh([-5:5])  InternalRulePriority=Speed  RndMeth=Simplest
  Clock : Clock
  Clock1 : Clock
  Constant : Constant  Value=simu.dt
  Constant1 : Constant  Value=10
  Constant2 : Constant  Value=0
  Constant3 : Constant  Value=0
  Constant4 : Constant  Value=R.WE_Mode
  Delay : Delay  DelayLength=1  InitialCondition=[R.WE_GearboxRatio, 0, R.WE_v0]'
  Delay1 : Delay  DelayLength=1  InitialCondition=diag([0.1, 0.1, 1])^2
  Delay2 : Delay  DelayLength=1  InitialCondition=zeros(3,1)
  Demux : Demux  Outputs=3
  Demux1 : Demux  Outputs=2
  Discrete Filter : DiscreteFilter  Numerator=F.F_WSEBlPitch.b  Denominator=F.F_WSEBlPitch.a
  Discrete Filter1 : DiscreteFilter  Numerator=F.HSS.b  Denominator=F.HSS.a  InitialStates=R.VS_RefSpd/(sum(F.HSS.a(2:end))+1)/R.GBRatio
  Discrete Filter2 : DiscreteFilter  Numerator=F.F_GenTq.b  Denominator=F.F_GenTq.a  InitialStates=R.VS_RtTq/(sum(F.F_GenTq.a(2:end))+1)
  Discrete Filter3 : DiscreteFilter  Numerator=F.Wind.b  Denominator=F.Wind.a  InitialStates=10
  MATLAB Function : MATLAB Function  TreatAsAtomicUnit=on
  NaN break : MATLAB Function  TreatAsAtomicUnit=on
  Soft Start : MATLAB Function  TreatAsAtomicUnit=on
  Sum : Sum
  Switch : Switch  Criteria=u2 > Threshold  Threshold=0.5  SaturateOnIntegerOverflow=off  InputSameDT=off
  Terminator : Terminator
  Terminator1 : Terminator
  Terminator2 : Terminator
  WE_Params : Subsystem
  WSE Inputs : Scope  NumInputPorts=3
  v_hat : Outport  VectorParamsAs1DForOutWhenUnconnected=off
  wires:
  MATLAB Function/2(xh) -> Delay/1
  Delay/1 -> Demux/1, MATLAB Function/6("xh ")
  MATLAB Function/3(P) -> Delay1/1
  Delay1/1 -> MATLAB Function/7("P ")
  omega_r/1 -> Discrete Filter1/1
  tau_g/1 -> Discrete Filter2/1
  MATLAB Function/4(K) -> Delay2/1
  Delay2/1 -> MATLAB Function/8("K ")
  Constant/1 -> MATLAB Function/9(dt)
  Demux/2 -> Sum/1
  Demux/3 -> Sum/2
  Demux/1 -> Terminator/1
  Sum/1 -> 1-D Lookup Table/1
  1-D Lookup Table/1 -> MATLAB Function/5(A_op)
  WE_Params/1(WE_Params) -> MATLAB Function/4(WE_params)
  Clock/1 -> Soft Start/3(time)
  Constant1/1 -> Soft Start/4(generic)
  Constant2/1 -> Soft Start/2(endTime)
  Constant3/1 -> Soft Start/1(startTime)
  MATLAB Function/1(vh) -> NaN break/1(u)
  Discrete Filter/1 -> WSE Inputs/3, MATLAB Function/3(beta)  "WE_b"
  Discrete Filter1/1 -> MATLAB Function/1(omega_r), WSE Inputs/1  "WE_w"
  Discrete Filter2/1 -> MATLAB Function/2(tau_g), WSE Inputs/2  "WE_t"
  PitComT/1 -> Discrete Filter/1
  Soft Start/1(out) -> Switch/1
  Switch/1 -> v_hat/1
  HorWindV/1 -> MATLAB Function/11(HorWind), Discrete Filter3/1
  Constant4/1 -> Switch/2
  MATLAB Function/5(Debug) -> Demux1/1
  Demux1/1 -> Terminator1/1  "WE_Cp"
  Demux1/2 -> Terminator2/1  "WE_D"
  Clock1/1 -> MATLAB Function/10(t)
  Discrete Filter3/1 -> Switch/3
  NaN break/1(y) -> Soft Start/5(actual)

== system ROSCO_v1/BldPitch Controller/Integral ==
  SpeedErr : Inport
  Gain : Inport  Port=2
  Min Pitch : Inport  Port=3
  Gain1 : Gain  Gain=simu.dt
  Maximum Pitch : Constant  Value=R.PC_MaxPit
  Minimum Pitch : Constant  Value=R.PC_MinPit
  Multiply : Product
  Saturate Integral Term : simulink/Discontinuities/Saturation Dynamic  OutMin=[]  OutMax=[]  OutDataTypeStr=Inherit: Same as second input  OutDataType=fixdt(1, 16)  OutScaling=2^-10  RndMeth=Nearest  DoSatur=off
  Sum : Sum  Inputs=|++
  Unit Delay : UnitDelay  SampleTime=-1  HasFrameUpgradeWarning=on
  IntSpdErr : Outport  VectorParamsAs1DForOutWhenUnconnected=off
  wires:
  Maximum Pitch/1 -> Saturate Integral Term/1
  Unit Delay/1 -> Sum/2
  Sum/1 -> Saturate Integral Term/2
  SpeedErr/1 -> Gain1/1
  Gain/1 -> Multiply/2
  Saturate Integral Term/1 -> IntSpdErr/1, Unit Delay/1
  Gain1/1 -> Multiply/1
  Multiply/1 -> Sum/1
  Min Pitch/1 -> Saturate Integral Term/3

== system ROSCO_v1/Fl_PD/Integral ==
  x : Inport
  Gain : Inport  Port=2
  Gain1 : Gain  Gain=simu.dt
  Maximum Pitch : Constant  Value=100
  Minimum Pitch : Constant  Value=-100
  Multiply : Product
  Saturate Integral Term : simulink/Discontinuities/Saturation Dynamic  OutMin=[]  OutMax=[]  OutDataTypeStr=Inherit: Same as second input  OutDataType=fixdt(1, 16)  OutScaling=2^-10  RndMeth=Nearest  DoSatur=off
  Scope : Scope  NumInputPorts=2
  Sum : Sum  Inputs=|++
  Unit Delay : UnitDelay  SampleTime=-1  HasFrameUpgradeWarning=on
  Int x : Outport  VectorParamsAs1DForOutWhenUnconnected=off
  wires:
  Maximum Pitch/1 -> Saturate Integral Term/1
  Unit Delay/1 -> Sum/2
  Minimum Pitch/1 -> Saturate Integral Term/3
  Sum/1 -> Saturate Integral Term/2
  x/1 -> Scope/1, Gain1/1
  Gain/1 -> Multiply/2
  Saturate Integral Term/1 -> Scope/2, Int x/1, Unit Delay/1
  Gain1/1 -> Multiply/1
  Multiply/1 -> Sum/1

== system ROSCO_v1/LinearModel_MATLABFcn/Extract Azimuth [deg] ==
  OutData : Inport
  Azimut : Scope  NumInputPorts=2
  Extract Azimuth : Fcn  Expr=u(strmatch('Azimuth',OutList))
  Extract RotSpeed : Fcn  Expr=u(strmatch('RotSpeed',OutList))
  Integrator : Integrator
  mod2pi : Fcn  Expr=rem(u, 2*pi)
  rad2deg : Gain  Gain=1/pi*180
  rpm2rad/s : Gain  Gain=pi/30
  Azimuth : Outport
  wires:
  Extract Azimuth/1 -> Azimut/1
  Extract RotSpeed/1 -> rpm2rad/s/1
  rad2deg/1 -> Azimuth/1, Azimut/2
  Integrator/1 -> mod2pi/1
  mod2pi/1 -> rad2deg/1
  rpm2rad/s/1 -> Integrator/1
  OutData/1 -> Extract Azimuth/1, Extract RotSpeed/1

== system ROSCO_v1/LinearModel_MATLABFcn/SwitchOP ==
  WindSpeed : Inport
  Constant : Constant  Value=StateSpace.B
  Constant1 : Constant  Value=StateSpace.A
  Constant2 : Constant  Value=StateSpace.yop_list
  Constant3 : Constant  Value=StateSpace.uop  VectorParams1D=off
  Constant5 : Constant  Value=StateSpace.D
  Constant6 : Constant  Value=StateSpace.C
  xdq_op : Constant  Value=StateSpace.xop
  A : Outport
  B : Outport  Port=2
  C : Outport  Port=3
  D : Outport  Port=4
  yop_list : Outport  Port=5
  xop : Outport  Port=6
  uop : Outport  Port=7
  wires:
  Constant5/1 -> D/1
  Constant/1 -> B/1
  Constant6/1 -> C/1
  Constant1/1 -> A/1
  Constant2/1 -> yop_list/1
  xdq_op/1 -> xop/1
  Constant3/1 -> uop/1

== system ROSCO_v1/LinearModel_MATLABFcn/y_NonLinear ==
  OutData : Inport
  Extract GenSpeed : Fcn  Expr=u(strmatch('GenSpeed',OutList))
  Extract RootMyc1 : Fcn  Expr=u(strmatch('RootMyc1',OutList))
  Extract RootMyc2 : Fcn  Expr=u(strmatch('RootMyc2',OutList))
  Extract RootMyc3 : Fcn  Expr=u(strmatch('RootMyc3',OutList))
  Extract RotSpeed : Fcn  Expr=u(strmatch('RotSpeed',OutList))
  Mux : Mux  Inputs=5
  y_NR : Outport
  wires:
  Extract RotSpeed/1 -> Mux/2
  Extract GenSpeed/1 -> Mux/1
  Extract RootMyc3/1 -> Mux/5
  Extract RootMyc2/1 -> Mux/4
  Mux/1 -> y_NR/1
  Extract RootMyc1/1 -> Mux/3
  OutData/1 -> Extract RootMyc1/1, Extract RootMyc3/1, Extract RootMyc2/1, Extract RotSpeed/1, Extract GenSpeed/1

== system ROSCO_v1/LinearModel_Simulink/Extract Azimuth [deg] ==
  OutData : Inport
  Azimut : Scope  NumInputPorts=2
  Extract Azimuth : Fcn  Expr=u(strmatch('Azimuth',OutList))
  Extract RotSpeed : Fcn  Expr=u(strmatch('RotSpeed',OutList))
  Integrator : Integrator
  mod2pi : Fcn  Expr=rem(u, 2*pi)
  rad2deg : Gain  Gain=1/pi*180
  rpm2rad/s : Gain  Gain=pi/30
  Azimuth : Outport
  wires:
  OutData/1 -> Extract RotSpeed/1, Extract Azimuth/1
  rpm2rad/s/1 -> Integrator/1
  mod2pi/1 -> rad2deg/1
  Integrator/1 -> mod2pi/1
  rad2deg/1 -> Azimut/2, Azimuth/1
  Extract RotSpeed/1 -> rpm2rad/s/1
  Extract Azimuth/1 -> Azimut/1

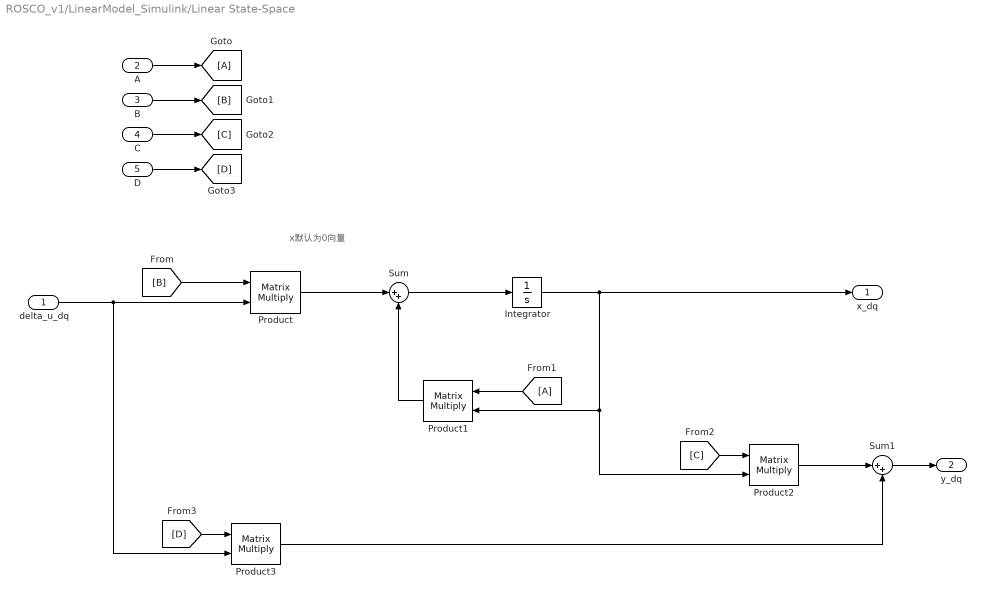
== system ROSCO_v1/LinearModel_Simulink/Linear State-Space ==
  note: x默认为0向量
  delta_u_dq : Inport
  A : Inport  Port=2
  B : Inport  Port=3
  C : Inport  Port=4
  D : Inport  Port=5
  From1 : From
  Goto : Goto
  Integrator : Integrator
  Product{,1..3} (4 alike) : Product  Multiplication=Matrix(*)
  Sum : Sum  Inputs=|++
  Sum1 : Sum  Inputs=|++
  x_dq : Outport
  y_dq : Outport  Port=2
  wires:
  delta_u_dq/1 -> Product3/2, Product/2
  Product/1 -> Sum/1
  Sum/1 -> Integrator/1
  Integrator/1 -> Product2/2, Product1/2, x_dq/1
  Product1/1 -> Sum/2
  Product2/1 -> Sum1/1
  Product3/1 -> Sum1/2
  Sum1/1 -> y_dq/1
  [B] -> Product/1
  From1/1 -> Product1/1
  [C] -> Product2/1
  [D] -> Product3/1
  A/1 -> Goto/1
  B/1 -> [B]
  C/1 -> [C]
  D/1 -> [D]

== system ROSCO_v1/LinearModel_Simulink/Switch op under Azimuth ==
  Azimuth : Inport
  delta_xdq : Inport  Port=2
  yop_list : Inport  Port=3
  xop : Inport  Port=4
  Integrator : Integrator
  Scope : Scope
  Select delta_wg : Fcn  Expr=u(11)
  Select wg : Fcn  Expr=u(11)
  Sum2 : Sum  Inputs=|++
  Switch op under Azimuth : MATLAB Function  TreatAsAtomicUnit=on
  "[deg]" : Constant  Value=Azimuth_list
  mod2pi : Fcn  Expr=rem(u, 2*pi)
  rad2deg : Gain  Gain=1/pi*180
  yop : Outport
  Azimuth_out : Outport  Port=2
  wires:
  "[deg]"/1 -> Switch op under Azimuth/2(Azimuth_list)
  Switch op under Azimuth/1(yop) -> yop/1
  Azimuth/1 -> Switch op under Azimuth/1(Azimuth)
  yop_list/1 -> Switch op under Azimuth/3(yop_36)
  rad2deg/1 -> Azimuth_out/1
  mod2pi/1 -> rad2deg/1
  Integrator/1 -> mod2pi/1
  Sum2/1 -> Integrator/1, Scope/1
  xop/1 -> Select wg/1
  delta_xdq/1 -> Select delta_wg/1
  Select delta_wg/1 -> Sum2/2
  Select wg/1 -> Sum2/1

== system ROSCO_v1/LinearModel_Simulink/SwitchOP ==
  WindSpeed : Inport
  Constant : Constant  Value=StateSpace.B
  Constant1 : Constant  Value=StateSpace.A
  Constant2 : Constant  Value=StateSpace.yop_list
  Constant3 : Constant  Value=StateSpace.uop  VectorParams1D=off
  Constant5 : Constant  Value=StateSpace.D
  Constant6 : Constant  Value=StateSpace.C
  MATLAB Function : MATLAB Function  TreatAsAtomicUnit=on
  xdq_op : Constant  Value=StateSpace.xop
  A : Outport
  B : Outport  Port=2
  C : Outport  Port=3
  D : Outport  Port=4
  yop_list : Outport  Port=5
  xop : Outport  Port=6
  uop : Outport  Port=7
  wires:
  Constant5/1 -> D/1
  Constant/1 -> B/1
  Constant6/1 -> C/1
  Constant1/1 -> A/1
  Constant2/1 -> yop_list/1
  xdq_op/1 -> xop/1
  Constant3/1 -> uop/1
  WindSpeed/1 -> MATLAB Function/1(u)

== system ROSCO_v1/LinearModel_Simulink/Transverseu ==
  Azimuth : Inport
  delta_u : Inport  Port=2
  new_seq_inp : Inport  Port=3
  Constant7 : Constant  Value=StateSpace.n_FixFrameInputs
  Constant8 : Constant  Value=StateSpace.n_RotTripletInputs
  MATLAB Function : MATLAB Function  TreatAsAtomicUnit=on
  delta_u_dq : Outport
  wires:
  Constant8/1 -> MATLAB Function/3(n_RotTripletInputs)
  Azimuth/1 -> MATLAB Function/1(Azimuth)
  Constant7/1 -> MATLAB Function/2(n_FixFrameInputs)
  delta_u/1 -> MATLAB Function/4(delta_u)
  new_seq_inp/1 -> MATLAB Function/5(new_seq_inp)
  MATLAB Function/1(delat_u_dq) -> delta_u_dq/1

== system ROSCO_v1/LinearModel_Simulink/y_NonLinear ==
  OutData : Inport
  Extract GenSpeed : Fcn  Expr=u(strmatch('GenSpeed',OutList))
  Extract RootMyc1 : Fcn  Expr=u(strmatch('RootMyc1',OutList))
  Extract RootMyc2 : Fcn  Expr=u(strmatch('RootMyc2',OutList))
  Extract RootMyc3 : Fcn  Expr=u(strmatch('RootMyc3',OutList))
  Extract RotSpeed : Fcn  Expr=u(strmatch('RotSpeed',OutList))
  Mux : Mux  Inputs=5
  y_NR : Outport
  wires:
  OutData/1 -> Extract GenSpeed/1, Extract RotSpeed/1, Extract RootMyc2/1, Extract RootMyc3/1, Extract RootMyc1/1
  Extract RootMyc1/1 -> Mux/3
  Mux/1 -> y_NR/1
  Extract RootMyc2/1 -> Mux/4
  Extract RootMyc3/1 -> Mux/5
  Extract GenSpeed/1 -> Mux/1
  Extract RotSpeed/1 -> Mux/2

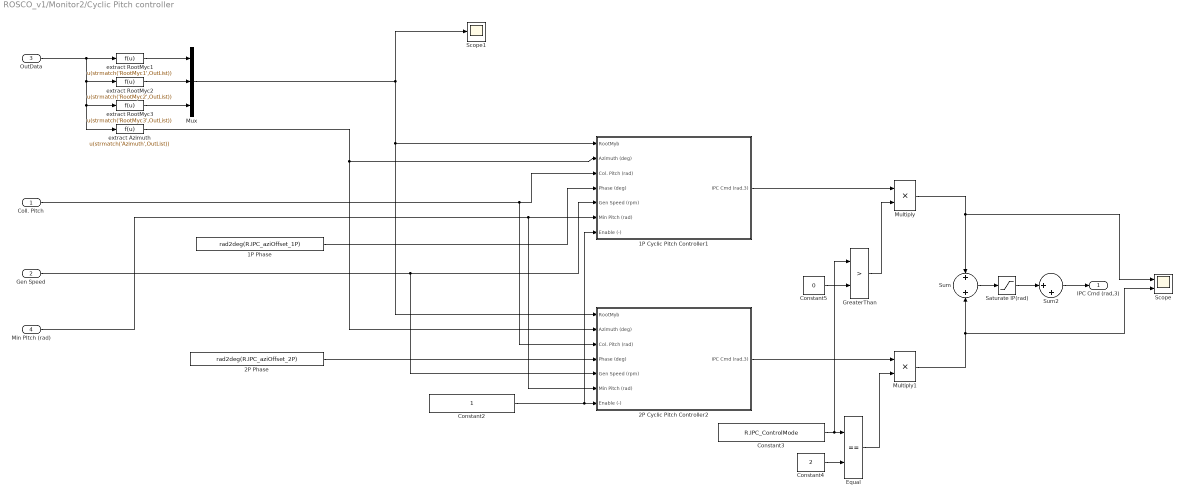
== system ROSCO_v1/Monitor2/Cyclic Pitch controller ==
  Coll. Pitch : Inport
  Gen Speed : Inport  Port=2
  OutData : Inport  Port=3
  Min PItch (rad) : Inport  Port=4
  1P Cyclic Pitch Controller1 : Subsystem
  1P Phase : Constant  Value=rad2deg(R.IPC_aziOffset_1P)
  2P Cyclic Pitch Controller2 : Subsystem
  2P Phase : Constant  Value=rad2deg(R.IPC_aziOffset_2P)
  Constant2 : Constant
  Constant3 : Constant  Value=R.IPC_ControlMode
  Constant4 : Constant  Value=2
  Constant5 : Constant  Value=0
  Equal : RelationalOperator  Operator===  OutDataTypeStr=boolean  RndMeth=Simplest  InputSameDT=off
  GreaterThan : RelationalOperator  Operator=>  OutDataTypeStr=boolean  RndMeth=Simplest  InputSameDT=off
  Multiply : Product
  Multiply1 : Product
  Mux : Mux  Inputs=3
  Saturate IP(rad) : Saturate  UpperLimit=0.052  LowerLimit=-0.052
  Scope : Scope  NumInputPorts=2
  Scope1 : Scope
  Sum : Sum  Inputs=+|+
  Sum2 : Sum  Inputs=|++
  extract Azimuth : Fcn  Expr=u(strmatch('Azimuth',OutList))
  extract RootMyc1 : Fcn  Expr=u(strmatch('RootMyc1',OutList))
  extract RootMyc2 : Fcn  Expr=u(strmatch('RootMyc2',OutList))
  extract RootMyc3 : Fcn  Expr=u(strmatch('RootMyc3',OutList))
  IPC Cmd (rad,3) : Outport  VectorParamsAs1DForOutWhenUnconnected=off
  wires:
  1P Phase/1 -> 1P Cyclic Pitch Controller1/4(Phase (deg))
  Coll. Pitch/1 -> 2P Cyclic Pitch Controller2/3(Col. Pitch (rad)), 1P Cyclic Pitch Controller1/3(Col. Pitch (rad))
  Gen Speed/1 -> 2P Cyclic Pitch Controller2/5(Gen Speed (rpm)), 1P Cyclic Pitch Controller1/5(Gen Speed (rpm))
  1P Cyclic Pitch Controller1/1(IPC Cmd (rad,3)) -> Multiply/1
  Mux/1 -> Scope1/1, 1P Cyclic Pitch Controller1/1(RootMyb), 2P Cyclic Pitch Controller2/1(RootMyb)
  extract Azimuth/1 -> 2P Cyclic Pitch Controller2/2(Azimuth (deg)), 1P Cyclic Pitch Controller1/2(Azimuth (deg))
  Min PItch (rad)/1 -> 2P Cyclic Pitch Controller2/6(Min Pitch (rad)), 1P Cyclic Pitch Controller1/6(Min Pitch (rad))
  2P Phase/1 -> 2P Cyclic Pitch Controller2/4(Phase (deg))
  2P Cyclic Pitch Controller2/1(IPC Cmd (rad,3)) -> Multiply1/1
  Multiply1/1 -> Scope/2, Sum/2
  Multiply/1 -> Sum/1, Scope/1
  Sum/1 -> Saturate IP(rad)/1
  Sum2/1 -> IPC Cmd (rad,3)/1
  Constant2/1 -> 1P Cyclic Pitch Controller1/7(Enable (-)), 2P Cyclic Pitch Controller2/7(Enable (-))
  Constant4/1 -> Equal/2
  Equal/1 -> Multiply1/2
  Constant3/1 -> GreaterThan/1, Equal/1
  Constant5/1 -> GreaterThan/2
  GreaterThan/1 -> Multiply/2
  extract RootMyc2/1 -> Mux/2
  extract RootMyc3/1 -> Mux/3
  OutData/1 -> extract RootMyc1/1, extract RootMyc2/1, extract Azimuth/1, extract RootMyc3/1
  extract RootMyc1/1 -> Mux/1
  Saturate IP(rad)/1 -> Sum2/1

== system ROSCO_v1/PitchSaturation/Integral ==
  x : Inport
  Gain : Inport  Port=2
  Gain1 : Gain  Gain=simu.dt
  Maximum Pitch : Constant  Value=100
  Minimum Pitch : Constant  Value=-100
  Multiply : Product
  Saturate Integral Term : simulink/Discontinuities/Saturation Dynamic  OutMin=[]  OutMax=[]  OutDataTypeStr=Inherit: Same as second input  OutDataType=fixdt(1, 16)  OutScaling=2^-10  RndMeth=Nearest  DoSatur=off
  Scope : Scope  NumInputPorts=2
  Sum : Sum  Inputs=|++
  Unit Delay : UnitDelay  SampleTime=-1  HasFrameUpgradeWarning=on
  Int x : Outport  VectorParamsAs1DForOutWhenUnconnected=off
  wires:
  Maximum Pitch/1 -> Saturate Integral Term/1
  Unit Delay/1 -> Sum/2
  Minimum Pitch/1 -> Saturate Integral Term/3
  Sum/1 -> Saturate Integral Term/2
  x/1 -> Scope/1, Gain1/1
  Gain/1 -> Multiply/2
  Saturate Integral Term/1 -> Scope/2, Int x/1, Unit Delay/1
  Gain1/1 -> Multiply/1
  Multiply/1 -> Sum/1

== system ROSCO_v1/SetpointSmoother/Filter Delta_GenRef ==
  GainBias : Inport
  Discrete Filter : DiscreteFilter  Numerator=F.F_SS.b  Denominator=F.F_SS.a
  GainBiasF : Outport  VectorParamsAs1DForOutWhenUnconnected=off
  wires:
  Discrete Filter/1 -> GainBiasF/1
  GainBias/1 -> Discrete Filter/1

== system ROSCO_v1/Torque Controller/Integral ==
  SpeedErr : Inport
  Gain : Inport  Port=2
  Gain1 : Gain  Gain=simu.dt
  Maximum Torque : Constant  Value=R.VS_RtTq
  Minimum Torque : Constant  Value=0
  Multiply : Product
  Saturate Integral Term : simulink/Discontinuities/Saturation Dynamic  OutMin=[]  OutMax=[]  OutDataTypeStr=Inherit: Same as second input  OutDataType=fixdt(1, 16)  OutScaling=2^-10  RndMeth=Nearest  DoSatur=off
  Sum : Sum  Inputs=|++
  Unit Delay : UnitDelay  InitialCondition=R.VS_RtTq  SampleTime=-1  HasFrameUpgradeWarning=on
  IntSpdErr : Outport  VectorParamsAs1DForOutWhenUnconnected=off
  wires:
  Maximum Torque/1 -> Saturate Integral Term/1
  Unit Delay/1 -> Sum/2
  Minimum Torque/1 -> Saturate Integral Term/3
  Sum/1 -> Saturate Integral Term/2
  SpeedErr/1 -> Gain1/1
  Gain/1 -> Multiply/2
  Saturate Integral Term/1 -> IntSpdErr/1, Unit Delay/1
  Gain1/1 -> Multiply/1
  Multiply/1 -> Sum/1

== system ROSCO_v1/Torque Controller/VS_OmegaRef ==
  WindSpeedEst : Inport
  Omega_opt : Subsystem
  Reference TSR : Constant  Value=R.VS_TSRopt
  Saturation : Saturate  UpperLimit=R.PC_RefSpd  LowerLimit=R.VS_MinOMSpd
  To Workspace1 : ToWorkspace  VariableName=Om_opt  SaveFormat=Timeseries  SampleTime=-1
  VS_OmegaOpt : Outport  VectorParamsAs1DForOutWhenUnconnected=off
  wires:
  WindSpeedEst/1 -> Omega_opt/2(Wind Speed)
  Omega_opt/1(Omega_opt) -> Saturation/1
  Reference TSR/1 -> Omega_opt/1(TSR_opt)
  Saturation/1 -> VS_OmegaOpt/1, To Workspace1/1

== system ROSCO_v1/Wind Speed Estimator/WE_Params ==
  Constant1 : Constant  Value=R.WE_Jtot
  Constant2 : Constant  Value=R.WE_RhoAir
  Constant3 : Constant  Value=R.WE_BladeRadius
  Constant4 : Constant  Value=R.WE_GearboxRatio
  Mux : Mux
  WE_Params : Outport
  wires:
  Constant2/1 -> Mux/2
  Mux/1 -> WE_Params/1
  Constant4/1 -> Mux/4
  Constant1/1 -> Mux/1
  Constant3/1 -> Mux/3

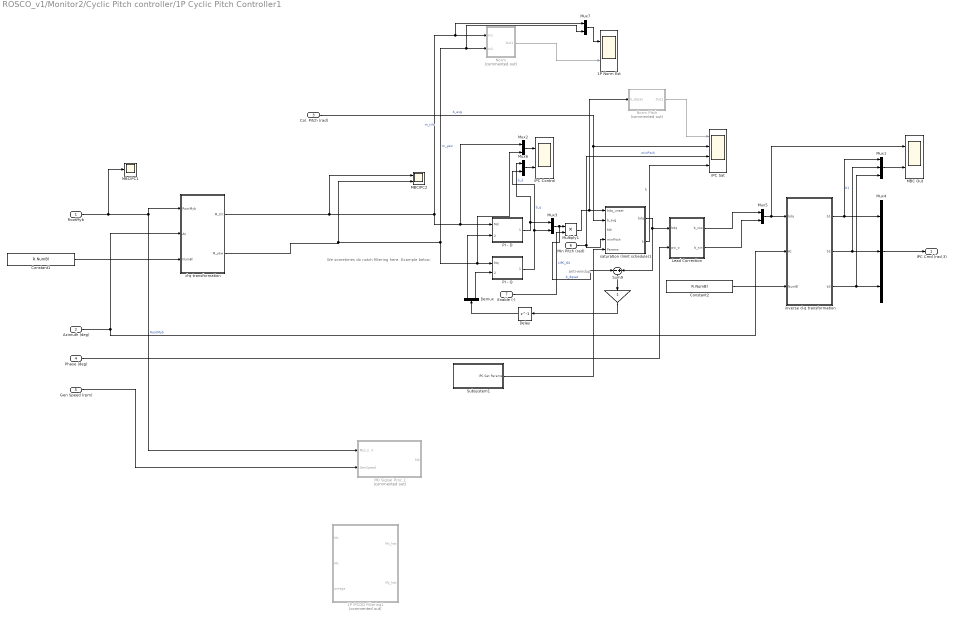
== system ROSCO_v1/Monitor2/Cyclic Pitch controller/1P Cyclic Pitch Controller1 ==
  note: We sometimes do notch filtering here. Example below.
  note: k
  note: anti-windup
  RootMyb : Inport
  Azimuth (deg) : Inport  Port=2
  Col. Pitch (rad) : Inport  Port=3
  Phase (deg) : Inport  Port=4
  Gen Speed (rpm) : Inport  Port=5
  Min Pitch (rad) : Inport  Port=6
  Enable (-) : Inport  Port=7
  " " : Gain
  1P IPCDQ Filtering1 : Subsystem  Commented=on
  1P Norm Est : Scope  NumInputPorts=2
  Constant1 : Constant  Value=R.NumBl
  Constant2 : Constant  Value=R.NumBl
  Delay : Delay  DelayLength=1
  Demux : Demux  Outputs=2
  IPC Control : Scope  NumInputPorts=2
  IPC Sat : Scope  NumInputPorts=4
  Lead Correction : MATLAB Function  TreatAsAtomicUnit=on
  M0 Signal Proc.1 : Subsystem  Commented=on
  MBC Out : Scope  NumInputPorts=2
  MBCIPC1 : Scope
  MBCIPC2 : Scope  NumInputPorts=2
  Multiply1 : Product
  Mux1 : Mux  Inputs=3
  Mux{2..3,5..7} (5 alike) : Mux  Inputs=2
  Mux4 : Mux  Inputs=3
  Norm : Subsystem  Commented=on
  Norm Pitch : Subsystem  Commented=on
  PI - D : Subsystem  TreatAsAtomicUnit=on  SystemSampleTime=simu.dt
      settings: MinAlgLoopOccurrences=on
  PI - Q : Subsystem  TreatAsAtomicUnit=on  SystemSampleTime=simu.dt
      settings: MinAlgLoopOccurrences=on
  Subsystem1 : Subsystem
  Sum9 : Sum  Inputs=-|+
  d-q transformation : MATLAB Function  TreatAsAtomicUnit=on
  inverse d-q transformation : MATLAB Function  TreatAsAtomicUnit=on
  saturation (limit schedule)1 : MATLAB Function  TreatAsAtomicUnit=on
  IPC Cmd (rad,3) : Outport  VectorParamsAs1DForOutWhenUnconnected=off
  wires:
  Col. Pitch (rad)/1 -> saturation (limit schedule)1/2(b_avg), IPC Sat/2  "b_avg"
  saturation (limit schedule)1/1(bdq) -> Sum9/2, Lead Correction/1(bdq)
  Gen Speed (rpm)/1 -> M0 Signal Proc.1/2(GenSpeed)
  d-q transformation/1(M_tilt) -> Mux2/1, PI - D/1(Md), Mux7/1, Norm/1(In1), MBCIPC2/1  "m_tilt"
  Mux5/1 -> MBC Out/1, inverse d-q transformation/1(bdq)
  inverse d-q transformation/3(b3) -> Mux1/3, Mux4/3
  Phase (deg)/1 -> Lead Correction/2(psi_o)
  PI - Q/1(Theta_yaw) -> Mux6/2, Mux3/2  "b_q"
  PI - D/1(Theta_tilt) -> Mux3/1, Mux6/1  "b_d"
  Demux/1 -> PI - D/2(Anti-windup)
  inverse d-q transformation/1(b1) -> Mux1/1, Mux4/1  "b1"
  Demux/2 -> PI - Q/2(Anti-windup)
  inverse d-q transformation/2(b2) -> Mux1/2, Mux4/2
  Mux4/1 -> IPC Cmd (rad,3)/1
  Delay/1 -> Demux/1
  " "/1 -> Delay/1
  RootMyb/1 -> M0 Signal Proc.1/1("My1,2, 3"), d-q transformation/1(RootMyb), MBCIPC1/1  "RootMyb"
  Sum9/1 -> " "/1
  Azimuth (deg)/1 -> d-q transformation/2(Az), inverse d-q transformation/2(Az)
  Lead Correction/1(b_cos) -> Mux5/1
  Lead Correction/2(b_sin) -> Mux5/2
  saturation (limit schedule)1/2(k) -> IPC Sat/4
  Constant1/1 -> d-q transformation/3(NumBl)
  Constant2/1 -> inverse d-q transformation/3(NumBl)
  d-q transformation/2(M_yaw) -> Mux2/2, PI - Q/1(Mq), Mux7/2, Norm/2(In2), MBCIPC2/2  "m_yaw"
  Mux1/1 -> MBC Out/2
  Mux6/1 -> IPC Control/2
  Mux2/1 -> IPC Control/1
  Mux7/1 -> 1P Norm Est/1
  Norm/1(Out1) -> 1P Norm Est/2
  Min Pitch (rad)/1 -> IPC Sat/3, saturation (limit schedule)1/4(minPitch)  "minPitch"
  Norm Pitch/1(Out1) -> IPC Sat/1
  Enable (-)/1 -> Multiply1/2  "cIPC_GS"
  Subsystem1/1(IPC Sat Params) -> saturation (limit schedule)1/5(Params)
  Mux3/1 -> Sum9/1, Multiply1/1  "b_dqsat"
  Multiply1/1 -> Norm Pitch/1(b_dqsat), saturation (limit schedule)1/1(bdq_unsat)
  ? -> 1P IPCDQ Filtering1/2(My)  "m_yaw"
